simulink model "distributed"  (Simulink 4.00)
settings: Solver=ode45  StartTime=0.0  StopTime=1  RelTol=1e-3
InitFcn:
  | clear functions
libraries: truetime x5
settings Model: Creator=anton  LastModifiedBy=anton  SaveTime=off  SaveOutput=off  UnconnectedInputMsg=none  UnconnectedOutputMsg=none  RTWOptions="-aEnforceIntegerDowncast=1 -aExtMode=0 -aFoldNonRolledExpr=1 -aForceParamTrailComments=0 -aGenerateComments=1 -aIgnoreCustomStorageClasses=0 -aIncHierarchyInIds=0 -aInlineInvariantSignals=0 -aLocalBlockOutputs=1 -aLogVarNameModifier=\"rt_\" -aRTWVerbose=1 -aRollThreshold=5 -aShowEliminatedStatements=1"  ExtModeAutoUpdateStatusClock=off  BlockReductionOpt=off

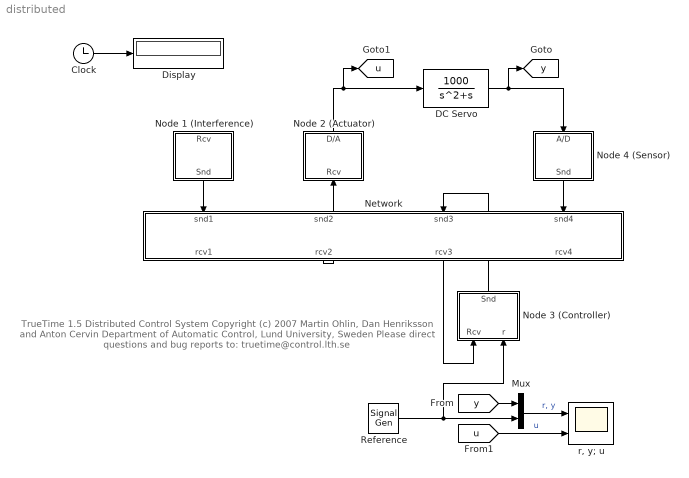
== system distributed ==
  note: TrueTime 1.5  Distributed Control System
      | Copyright (c) 2007
      | Martin Ohlin, Dan Henriksson and Anton Cervin
      | Department of Automatic Control, Lund University, Sweden
      | Please direct questions and bug reports to:  truetime@control.lth.se
  Clock : Clock
      settings: DisplayTime=off  Decimation=10
  DC Servo : TransferFcn  Numerator=[1000]  Denominator=[1 1 0]  AbsoluteTolerance=auto  Realization=auto
  Display : Display
      settings: Format=short
  Mux : Mux  Inputs=2
  Network : Subsystem  Orientation=down
      settings: RTWFcnNameOpts=Auto  RTWFileNameOpts=Auto
  Node 1 (Interference) : Subsystem  Orientation=down
      settings: RTWFcnNameOpts=Auto  RTWFileNameOpts=Auto
  Node 2 (Actuator) : Subsystem  Orientation=up
      settings: RTWFcnNameOpts=Auto  RTWFileNameOpts=Auto
  Node 3 (Controller) : Subsystem  Orientation=up
      settings: RTWFcnNameOpts=Auto  RTWFileNameOpts=Auto
  Node 4 (Sensor) : Subsystem  Orientation=down
      settings: RTWFcnNameOpts=Auto  RTWFileNameOpts=Auto
  Reference : SignalGenerator  WaveForm=square  Amplitude=1  Frequency=2  Units=Hertz
  "r, y; u" : Scope  NumInputPorts=2
      settings: TimeRange=1  YMin=-2~-5  YMax=2~5  SaveToWorkspace=off  SaveName=y  MaxDataPoints=5000
  tag scope: u=global, y=global
  wires:
  Clock/1 -> Display/1
  Network/2(rcv2) -> Node 2 (Actuator)/1(Rcv)
  Node 2 (Actuator)/1(D/A) -> DC Servo/1, [u]
  Node 4 (Sensor)/1(Snd) -> Network/4(snd4)
  DC Servo/1 -> Node 4 (Sensor)/1(A/D), [y]
  Node 3 (Controller)/1(Snd) -> Network/3(snd3)
  Mux/1 -> "r, y; u"/1  "r, y"
  [y] -> Mux/1
  Reference/1 -> Mux/2, Node 3 (Controller)/2(r)
  [u] -> "r, y; u"/2  "u"
  Node 1 (Interference)/1(Snd) -> Network/1(snd1)
  Network/3(rcv3) -> Node 3 (Controller)/1(Rcv)

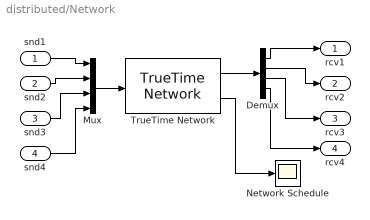
== system distributed/Network ==
  snd1 : Inport  Port=1  LatchInput=off
  snd2 : Inport  Port=2  LatchInput=off
  snd3 : Inport  Port=3  LatchInput=off
  snd4 : Inport  Port=4  LatchInput=off
  Demux : Demux  Outputs=4  BusSelectionMode=off
  Mux : Mux  Inputs=4
  Network Schedule : Scope
      settings: TimeRange=1  YMin=1  YMax=5  SaveToWorkspace=off  SaveName=nschedule  MaxDataPoints=5000
  TrueTime Network : truetime/TrueTime Network  nwtype=CSMA/AMP (CAN)  nwnbr=1  nnodes=4  rate=80000  minsize=40  lossprob=0  bandwidths=1  slotsize=20  schedule="[1 2 3  3 3 3]"  memsize=10000  buftype=Common buffer  overflow=Retransmit
  rcv1 : Outport  Port=1
  rcv2 : Outport  Port=2
  rcv3 : Outport  Port=3
  rcv4 : Outport  Port=4
  wires:
  Demux/1 -> rcv1/1
  Demux/2 -> rcv2/1
  Mux/1 -> TrueTime Network/1
  snd1/1 -> Mux/1
  snd2/1 -> Mux/2
  snd3/1 -> Mux/3
  Demux/3 -> rcv3/1
  snd4/1 -> Mux/4
  Demux/4 -> rcv4/1
  TrueTime Network/1 -> Demux/1
  TrueTime Network/2 -> Network Schedule/1

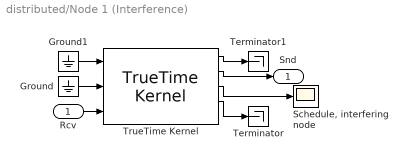
== system distributed/Node 1 (Interference) ==
  Rcv : Inport  Port=1  LatchInput=off
  Ground : Ground
  Ground1 : Ground
  "Schedule, interfering node" : Scope
      settings: TickLabels=on  TimeRange=2  YMin=0.5  YMax=2  SaveToWorkspace=off  SaveName=ScopeData  DataFormat=Array  MaxDataPoints=5000
  Terminator : Terminator
  Terminator1 : Terminator
  TrueTime Kernel : truetime/TrueTime Kernel  sfun=interference_init  args=0  battery=off  clockdrift=0  clockoffset=0
  Snd : Outport  Port=1
  wires:
  TrueTime Kernel/3 -> "Schedule, interfering node"/1
  TrueTime Kernel/2 -> Snd/1
  TrueTime Kernel/1 -> Terminator1/1
  Ground/1 -> TrueTime Kernel/2
  Rcv/1 -> TrueTime Kernel/3
  Ground1/1 -> TrueTime Kernel/1
  TrueTime Kernel/4 -> Terminator/1

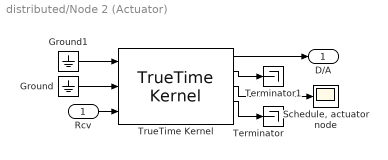
== system distributed/Node 2 (Actuator) ==
  Rcv : Inport  Port=1  LatchInput=off
  Ground : Ground
  Ground1 : Ground
  "Schedule, actuator node" : Scope
      settings: TickLabels=on  TimeRange=0.6  YMin=0.8  YMax=3.7  SaveToWorkspace=off  SaveName=ScopeData  DataFormat=Array  MaxDataPoints=5000
  Terminator : Terminator
  Terminator1 : Terminator
  TrueTime Kernel : truetime/TrueTime Kernel  sfun=actuator_init  args=0  battery=off  clockdrift=0  clockoffset=0
  D/A : Outport  Port=1
  wires:
  Ground1/1 -> TrueTime Kernel/1
  Rcv/1 -> TrueTime Kernel/3
  Ground/1 -> TrueTime Kernel/2
  TrueTime Kernel/1 -> D/A/1
  TrueTime Kernel/2 -> Terminator1/1
  TrueTime Kernel/3 -> "Schedule, actuator node"/1
  TrueTime Kernel/4 -> Terminator/1

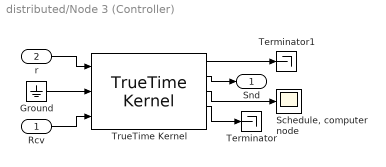
== system distributed/Node 3 (Controller) ==
  Rcv : Inport  Port=1  LatchInput=off
  r : Inport  Port=2  LatchInput=off
  Ground : Ground
  "Schedule, computer node" : Scope
      settings: TimeRange=0.6  YMin=0.8  YMax=4.7  SaveName=schedule  MaxDataPoints=5000
  Terminator : Terminator
  Terminator1 : Terminator
  TrueTime Kernel : truetime/TrueTime Kernel  sfun=controller_init  args=0  battery=off  clockdrift=0  clockoffset=0
  Snd : Outport  Port=1
  wires:
  TrueTime Kernel/2 -> Snd/1
  Ground/1 -> TrueTime Kernel/2
  r/1 -> TrueTime Kernel/1
  Rcv/1 -> TrueTime Kernel/3
  TrueTime Kernel/3 -> "Schedule, computer node"/1
  TrueTime Kernel/1 -> Terminator1/1
  TrueTime Kernel/4 -> Terminator/1

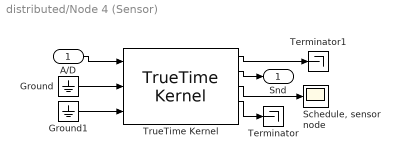
== system distributed/Node 4 (Sensor) ==
  A/D : Inport  Port=1  LatchInput=off
  Ground : Ground
  Ground1 : Ground
  "Schedule, sensor node" : Scope
      settings: TickLabels=on  TimeRange=0.6  YMin=0.8  YMax=3.7  SaveToWorkspace=off  SaveName=ScopeData  DataFormat=Array  MaxDataPoints=5000
  Terminator : Terminator
  Terminator1 : Terminator
  TrueTime Kernel : truetime/TrueTime Kernel  sfun=sensor_init  args=0  battery=off  clockdrift=0  clockoffset=0
  Snd : Outport  Port=1
  wires:
  TrueTime Kernel/4 -> Terminator/1
  TrueTime Kernel/3 -> "Schedule, sensor node"/1
  TrueTime Kernel/2 -> Snd/1
  TrueTime Kernel/1 -> Terminator1/1
  Ground/1 -> TrueTime Kernel/2
  Ground1/1 -> TrueTime Kernel/3
  A/D/1 -> TrueTime Kernel/1
